simulink model "Lab1_KF_LQR"  (R2019a)
settings: Solver=FixedStepAuto  StartTime=0.0  StopTime=10.0  RelTol=1e-3
undefined symbols (not defined in the file or in its folder): A, B, C, Klqr, Q_kf, R_kf
libraries: cstblocks x1
settings Model: Creator=emma  LastModifiedBy=emma

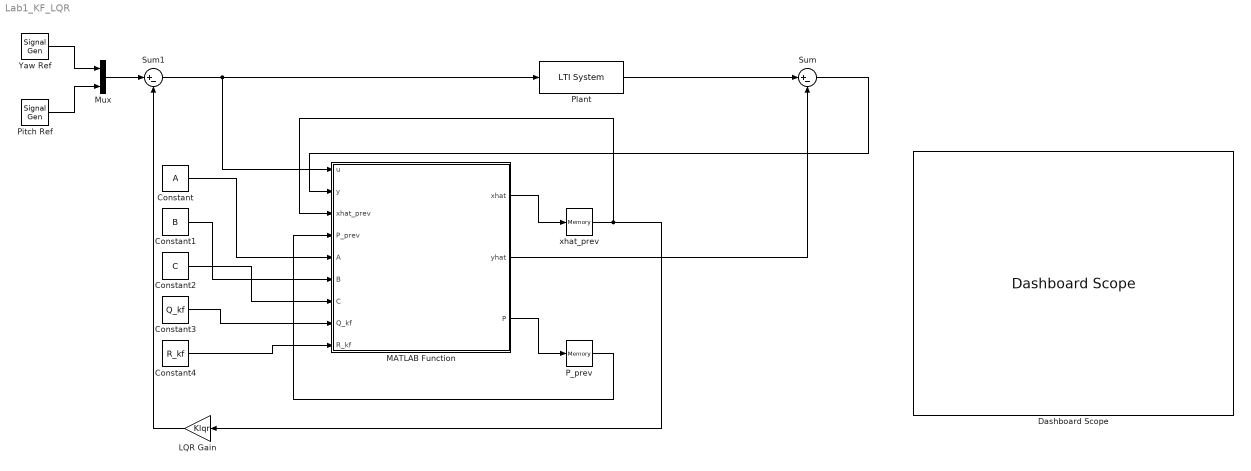
== system Lab1_KF_LQR ==
  Constant : Constant  Value=A
  Constant1 : Constant  Value=B
  Constant2 : Constant  Value=C
  Constant3 : Constant  Value=Q_kf  VectorParams1D=off
  Constant4 : Constant  Value=R_kf  VectorParams1D=off
  Dashboard Scope : DashboardScope
  LQR Gain : Gain  Gain=Klqr
  MATLAB Function : MATLAB Function  TreatAsAtomicUnit=on
  Mux : Mux  Inputs=2
  P_prev : Memory  InitialCondition=zeros(4,4)
  Pitch Ref : SignalGenerator  WaveForm=square  Amplitude=pi/6  Frequency=0.4  Units=rad/sec
  Plant : cstblocks/LTI System  sys=Gnom  IC=[]
  Sum : Sum  Inputs=|+-
  Sum1 : Sum  Inputs=|+-
  Yaw Ref : SignalGenerator  WaveForm=square  Amplitude=pi/4  Frequency=0.5  Units=rad/sec
  xhat_prev : Memory  InitialCondition=zeros(4,1)
  wires:
  Yaw Ref/1 -> Mux/1
  Pitch Ref/1 -> Mux/2
  xhat_prev/1 -> MATLAB Function/3(xhat_prev), LQR Gain/1
  P_prev/1 -> MATLAB Function/4(P_prev)
  Constant/1 -> MATLAB Function/5(A)
  Constant1/1 -> MATLAB Function/6(B)
  Constant2/1 -> MATLAB Function/7(C)
  Constant3/1 -> MATLAB Function/8(Q_kf)
  Constant4/1 -> MATLAB Function/9(R_kf)
  MATLAB Function/1(xhat) -> xhat_prev/1
  Mux/1 -> Sum1/1
  Sum/1 -> MATLAB Function/2(y)
  MATLAB Function/3(P) -> P_prev/1
  MATLAB Function/2(yhat) -> Sum/2
  LQR Gain/1 -> Sum1/2
  Sum1/1 -> Plant/1, MATLAB Function/1(u)
  Plant/1 -> Sum/1

== matlab function Lab1_KF_LQR/MATLAB Function ==
  data: u input; xhat output; y input; xhat_prev input; P_prev input; A input; B input; C input; Q_kf input; R_kf input; yhat output; P output
function [xhat,yhat,P] = kalman_wtf(u,y,xhat_prev,P_prev,A,B,C,Q_kf,R_kf)
    %kalman_wtf calculates the state estimate using the Kalman filter algorithm
    
    % prediction step
    xhat_est = A * xhat_prev + B * u ; % (4x4)*(4x1) + (4x2)*(2x1)
    P_est = A * P_prev * A' + Q_kf ; % (4x4)*(4,4)*(4x4)
    
    % update step
    K = (P_est * C')*inv(C * P_est * C' + R_kf) ; %(4x4)*(4*2)*((2x4)*(4x4)*(4x2) + (2,2))^-1
    xhat = xhat_est + K * (y - C * xhat_est) ; % (4x1) + (4x2)*((2x1) - (2x4)*(4x1))
    P = (eye(4) - K * C) * P_est ; % ((?) - (4x2)*(2x4))*(4x4)
    yhat = C * xhat ; 
end
